simulink model "airspeed_from_pitch_loop"  (R2016b)
settings: Solver=VariableStepAuto  StartTime=0.0  StopTime=10.0  RelTol=1e-3
undefined symbols (not defined in the file): a_theta1, a_theta2, a_theta3, a_V1, k_d_theta, k_i_v2, k_p_theta, k_p_v2, K_theta_DC, P
settings Model: Creator=geun2  LastModifiedBy=geun2

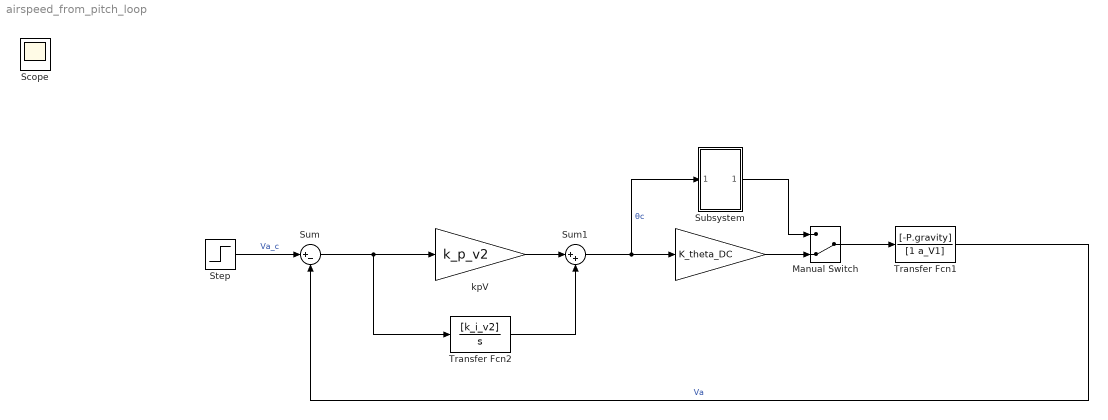
== system airspeed_from_pitch_loop ==
  " " : Gain  Gain=K_theta_DC
  Manual Switch : ManualSwitch  CurrentSetting=0
  Step : Step  SampleTime=0
  Subsystem : Subsystem
  Sum : Sum  Inputs=|+-
  Sum1 : Sum  Inputs=|++
  Transfer Fcn1 : TransferFcn  Numerator=[-P.gravity]  Denominator=[1 a_V1]
  Transfer Fcn2 : TransferFcn  Numerator=[k_i_v2]  Denominator=[1 0]
  kpV : Gain  Gain=k_p_v2
  Scope : Scope
  wires:
  Sum/1 -> Transfer Fcn2/1, kpV/1
  Transfer Fcn1/1 -> Sum/2  "Va"
  Step/1 -> Sum/1  "Va_c"
  kpV/1 -> Sum1/1
  Transfer Fcn2/1 -> Sum1/2
  Sum1/1 -> " "/1, Subsystem/1(In1)  "θc"
  Manual Switch/1 -> Transfer Fcn1/1
  " "/1 -> Manual Switch/2
  Subsystem/1(Out1) -> Manual Switch/1

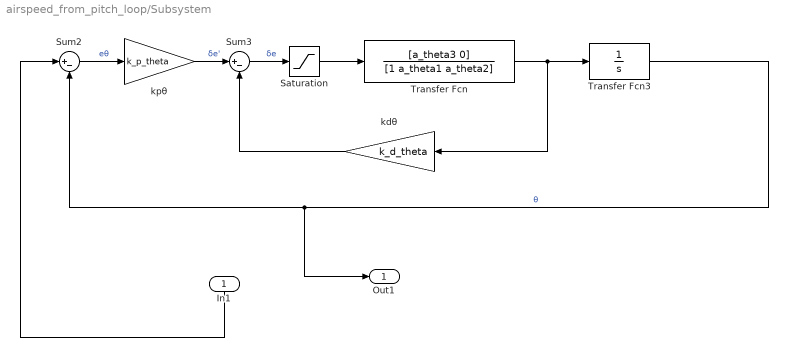
== system airspeed_from_pitch_loop/Subsystem ==
  In1 : Inport
  Saturation : Saturate  UpperLimit=45*pi/180  LowerLimit=-45*pi/180
  Sum2 : Sum  Inputs=|+-
  Sum3 : Sum  Inputs=|+-
  Transfer Fcn : TransferFcn  Numerator=[a_theta3 0]  Denominator=[1 a_theta1 a_theta2]
  Transfer Fcn3 : TransferFcn  Denominator=[1 0]
  kdθ : Gain  Gain=k_d_theta
  kpθ : Gain  Gain=k_p_theta
  Out1 : Outport
  wires:
  Sum2/1 -> kpθ/1  "eθ"
  kpθ/1 -> Sum3/1  "δe'"
  Sum3/1 -> Saturation/1  "δe"
  Transfer Fcn/1 -> Transfer Fcn3/1, kdθ/1
  Transfer Fcn3/1 -> Out1/1, Sum2/2  "θ"
  kdθ/1 -> Sum3/2
  Saturation/1 -> Transfer Fcn/1
  In1/1 -> Sum2/1
